simulink model "BWmodle"  (R2024a)
settings: Solver=ode4  StartTime=0  StopTime=10  FixedStep=1e-4  MaxStep=1e-4  RelTol=1e-3
settings Model: Creator=ch854  LastModifiedBy=18311
settings SolverCC: ZeroCrossAlgorithm=Adaptive
settings RTWCC: GPUComputeCapability=3.5

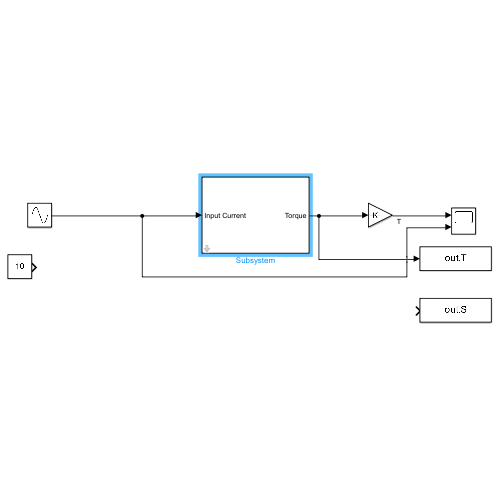
[thumbnail: Simulink's stored preview of the top-level diagram]
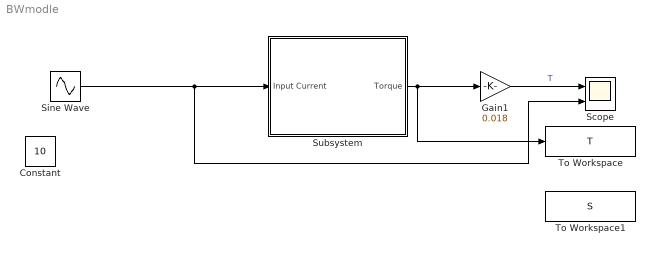
== system BWmodle ==
  Constant : Constant  Value=10
  Gain1 : Gain  Gain=0.018
  Scope : Scope  NumInputPorts=2
  Sine Wave : Sin  Amplitude=5  Bias=5  Frequency=pi*4  SampleTime=0
  Subsystem : Subsystem  mask{c=-2, k=58.857, d=0.6, alpha=-37.209}
  To Workspace : ToWorkspace  VariableName=T  SampleTime=-1
  To Workspace1 : ToWorkspace  VariableName=S  SampleTime=-1
  wires:
  Gain1/1 -> Scope/1  "T"
  Subsystem/1(Torque) -> Gain1/1, To Workspace/1
  Sine Wave/1 -> Scope/2, Subsystem/1(Input Current)

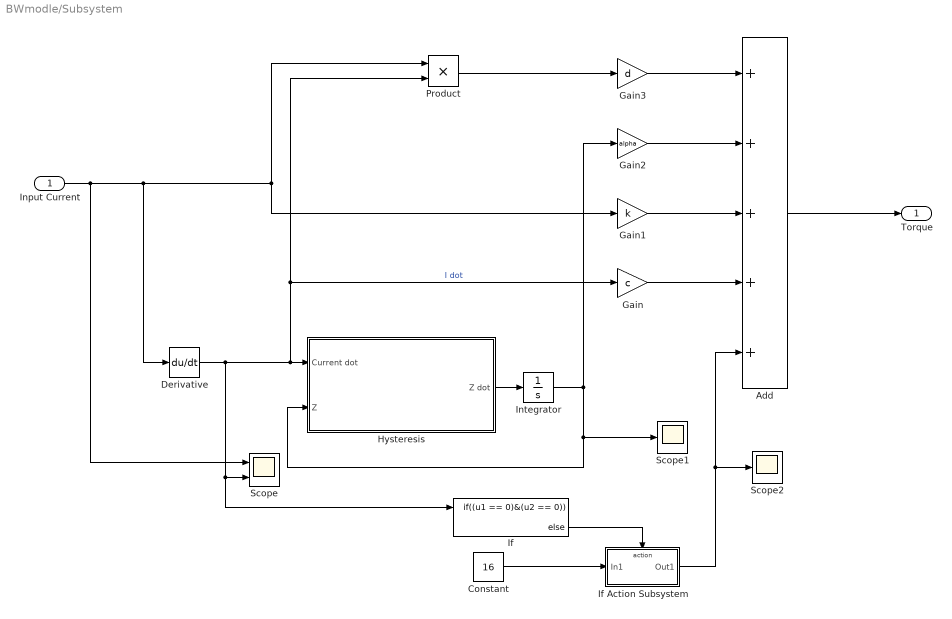
== system BWmodle/Subsystem ==
  Input Current : Inport
  Add : Sum  Inputs=+++++
  Constant : Constant  Value=16
  Derivative : Derivative
  Gain : Gain  Gain=c
  Gain1 : Gain  Gain=k
  Gain2 : Gain  Gain=alpha
  Gain3 : Gain  Gain=d
  Hysteresis : Subsystem  mask{theta=-0.41731, beta=-0.83796, v=2.2221, gamma=2.0211}
  If : If  NumInputs=2  IfExpression=(u1 == 0)&(u2 == 0)
  If Action Subsystem : Subsystem  TreatAsAtomicUnit=on
  Integrator : Integrator
  Product : Product
  Scope : Scope  NumInputPorts=2
  Scope1 : Scope
  Scope2 : Scope
  Torque : Outport
  wires:
  Derivative/1 -> Hysteresis/1(Current dot), Product/2, Gain/1, Scope/2, If/1  "I dot"
  Gain/1 -> Add/4
  Gain1/1 -> Add/3
  Gain2/1 -> Add/2
  Gain3/1 -> Add/1
  Product/1 -> Gain3/1
  Input Current/1 -> Scope/1, Derivative/1, Product/1, Gain1/1
  Integrator/1 -> Scope1/1, Hysteresis/2(Z), Gain2/1
  Hysteresis/1(Z dot) -> Integrator/1
  Add/1 -> Torque/1
  Constant/1 -> If Action Subsystem/1(In1)
  If Action Subsystem/1(Out1) -> Scope2/1, Add/5
  If/2 -> If Action Subsystem/Action

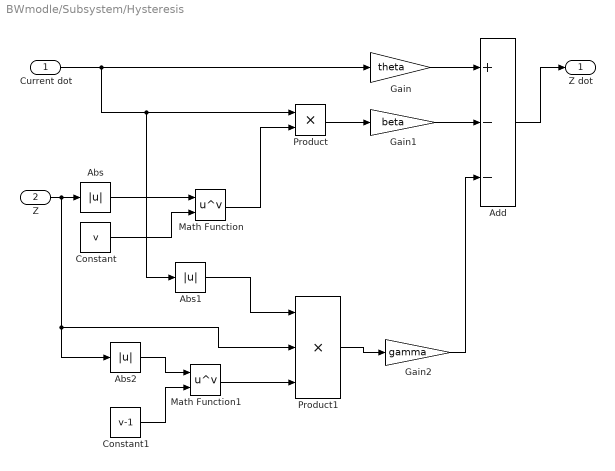
== system BWmodle/Subsystem/Hysteresis ==
  Current dot : Inport
  Z : Inport  Port=2
  Abs : Abs  SaturateOnIntegerOverflow=off
  Abs1 : Abs  SaturateOnIntegerOverflow=off
  Abs2 : Abs  SaturateOnIntegerOverflow=off
  Add : Sum  Inputs=+--
  Constant : Constant  Value=v
  Constant1 : Constant  Value=v-1
  Gain : Gain  Gain=theta
  Gain1 : Gain  Gain=beta
  Gain2 : Gain  Gain=gamma
  Math Function : Math  Operator=pow
  Math Function1 : Math  Operator=pow
  Product : Product
  Product1 : Product  Inputs=3
  Z dot : Outport
  wires:
  Current dot/1 -> Abs1/1, Product/1, Gain/1
  Gain/1 -> Add/1
  Z/1 -> Product1/2, Abs2/1, Abs/1
  Math Function/1 -> Product/2
  Product/1 -> Gain1/1
  Gain1/1 -> Add/2
  Math Function1/1 -> Product1/3
  Abs1/1 -> Product1/1
  Add/1 -> Z dot/1
  Abs/1 -> Math Function/1
  Constant/1 -> Math Function/2
  Product1/1 -> Gain2/1
  Gain2/1 -> Add/3
  Abs2/1 -> Math Function1/1
  Constant1/1 -> Math Function1/2

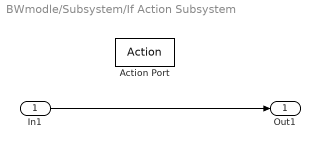
== system BWmodle/Subsystem/If Action Subsystem ==
  In1 : Inport
  Action Port : ActionPort  ActionPortLabel=else
  Out1 : Outport
  wires:
  In1/1 -> Out1/1
